simulink model "model_2"  (R2019b)
settings: Solver=VariableStepAuto  StartTime=0.0  StopTime=30.0  RelTol=1e-3
values from neighbouring files (symbols this model uses):
  k = 5    [skrypt_2.m]
  kd = (2*w*T-1)/k    (= 4.82654824574)    [skrypt_2.m]
  kp = (w^2*T)/k    (= 10.5275780278)    [skrypt_2.m]
  T = 3    [skrypt_2.m]
  w = 2*pi/a    (= 4.18879020479)    [skrypt_2.m]
settings Model: Creator=szymo  LastModifiedBy=szymo

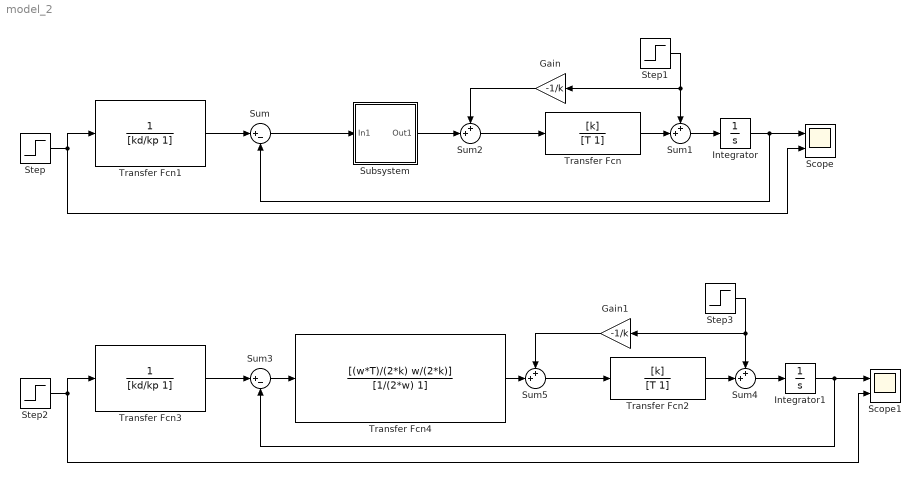
== system model_2 ==
  Gain : Gain  Gain=-1/k
  Gain1 : Gain  Gain=-1/k
  Integrator : Integrator
  Integrator1 : Integrator
  Scope : Scope  NumInputPorts=2
  Scope1 : Scope  NumInputPorts=2
  Step : Step  SampleTime=0
  Step1 : Step  After=3  SampleTime=0
  Step2 : Step  SampleTime=0
  Step3 : Step  After=3  SampleTime=0
  Subsystem : Subsystem
  Sum : Sum  Inputs=|+-
  Sum{1..2,4..5} (4 alike) : Sum  Inputs=++|
  Sum3 : Sum  Inputs=|+-
  Transfer Fcn : TransferFcn  Numerator=[k]  Denominator=[T 1]
  Transfer Fcn1 : TransferFcn  Denominator=[kd/kp 1]
  Transfer Fcn2 : TransferFcn  Numerator=[k]  Denominator=[T 1]
  Transfer Fcn3 : TransferFcn  Denominator=[kd/kp 1]
  Transfer Fcn4 : TransferFcn  Numerator=[(w*T)/(2*k) w/(2*k)]  Denominator=[1/(2*w) 1]
  wires:
  Step/1 -> Transfer Fcn1/1, Scope/2
  Sum/1 -> Subsystem/1(In1)
  Integrator/1 -> Sum/2, Scope/1
  Sum1/1 -> Integrator/1
  Transfer Fcn/1 -> Sum1/2
  Step1/1 -> Sum1/1, Gain/1
  Subsystem/1(Out1) -> Sum2/2
  Sum2/1 -> Transfer Fcn/1
  Gain/1 -> Sum2/1
  Transfer Fcn1/1 -> Sum/1
  Transfer Fcn3/1 -> Sum3/1
  Sum4/1 -> Integrator1/1
  Step3/1 -> Sum4/1, Gain1/1
  Gain1/1 -> Sum5/1
  Step2/1 -> Transfer Fcn3/1, Scope1/2
  Integrator1/1 -> Sum3/2, Scope1/1
  Sum3/1 -> Transfer Fcn4/1
  Sum5/1 -> Transfer Fcn2/1
  Transfer Fcn2/1 -> Sum4/2
  Transfer Fcn4/1 -> Sum5/2

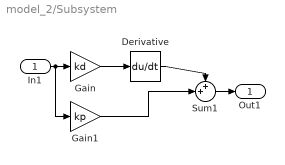
== system model_2/Subsystem ==
  In1 : Inport
  Derivative : Derivative
  Gain : Gain  Gain=kd
  Gain1 : Gain  Gain=kp
  Sum1 : Sum  Inputs=++|
  Out1 : Outport
  wires:
  Gain1/1 -> Sum1/2
  Gain/1 -> Derivative/1
  Derivative/1 -> Sum1/1
  In1/1 -> Gain1/1, Gain/1
  Sum1/1 -> Out1/1
